simulink model "V4_Modell_Wagen"  (R2022a)
settings: Solver=ode3  StartTime=0.0  StopTime=Zeit(end)  FixedStep=0.00001  RelTol=1e-3
values from neighbouring files (symbols this model uses):
  A = 0.01155    [V4_Parameter_Wagen_St.m]    (also in V4_Parameter_Wagen_Te.m; V4_Parameter_komplett_St.m; V4_Parameter_komplett_Te.m)
  c_W = 0.81    [V4_Parameter_Wagen_St.m]    (also in V4_Parameter_Wagen_Te.m; V4_Parameter_komplett_St.m; V4_Parameter_komplett_Te.m)
  g = 9.81    [V4_Parameter_Wagen_St.m]    (also in V4_Parameter_Wagen_Te.m; V4_Parameter_komplett_St.m; V4_Parameter_komplett_Te.m)
  gamma_rad = gamma_deg * (pi/180)    (= 0.349065850399)    [V4_Parameter_Wagen_St.m]    (also in V4_Parameter_Wagen_Te.m; V4_Parameter_komplett_St.m; V4_Parameter_komplett_Te.m)
  k = (m_Trans + m_ErsatzAntrieb + m_ErsatzRad) / (m_Trans)    [V4_Parameter_Wagen_St.m]    (also in V4_Parameter_Wagen_Te.m; V4_Parameter_komplett_St.m; V4_Parameter_komplett_Te.m)
  k_M = -0.038462    [V4_Parameter_EM.m]    (also in V4_Parameter_Wagen_St.m; V4_Parameter_Wagen_Te.m; V4_Parameter_komplett_St.m; V4_Parameter_komplett_Te.m)
  m_Trans = m_W + 4*m_R    (= 2.157)    [V4_Parameter_Wagen_St.m]    (also in V4_Parameter_Wagen_Te.m = 1.7232; V4_Parameter_komplett_St.m; V4_Parameter_komplett_Te.m = 1.7232)
  mu_R = 0.043    [V4_Parameter_Wagen_St.m]    (also in V4_Parameter_Wagen_Te.m = 0.045; V4_Parameter_komplett_St.m; V4_Parameter_komplett_Te.m = 0.045)
  r_ZR = 25 * (10^(-3))    (= 0.025)    [V4_Parameter_EM.m]    (also in V4_Parameter_Wagen_St.m = 0.021; V4_Parameter_Wagen_Te.m = 0.021; V4_Parameter_komplett_St.m; V4_Parameter_komplett_Te.m)
  rho_L = 1.2    [V4_Parameter_Wagen_St.m]    (also in V4_Parameter_Wagen_Te.m; V4_Parameter_komplett_St.m; V4_Parameter_komplett_Te.m)
settings Model: Creator=bornk  LastModifiedBy=bornk

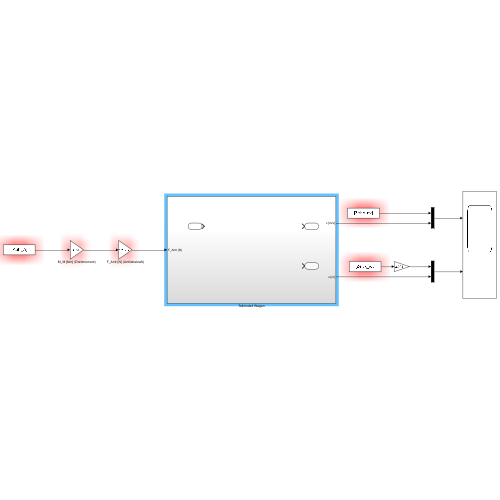
[thumbnail: Simulink's stored preview of the top-level diagram]
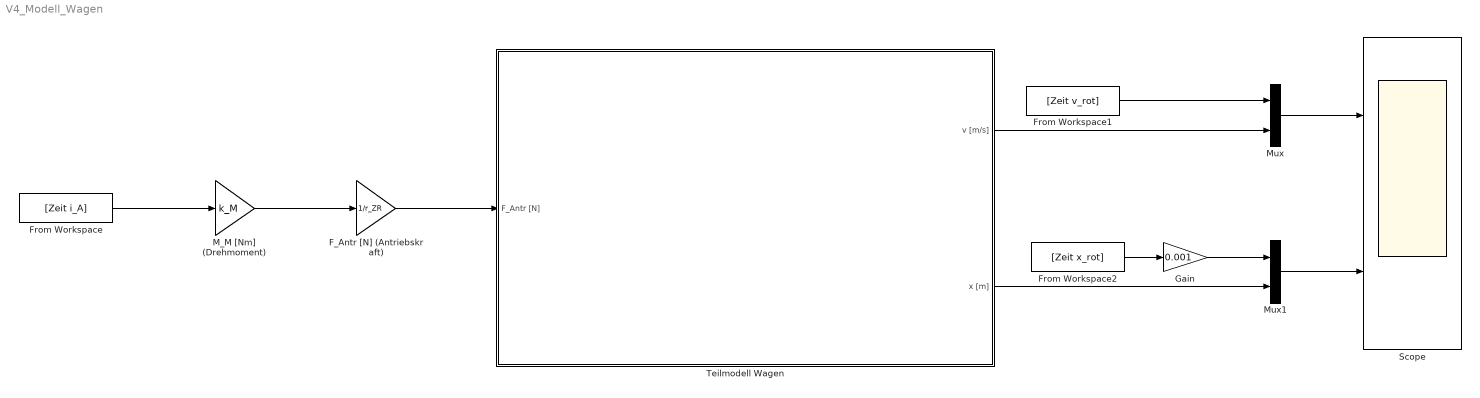
== system V4_Modell_Wagen ==
  F_Antr [N] (Antriebskraft) : Gain  Gain=1/r_ZR
  From Workspace : FromWorkspace  VariableName=[Zeit i_A]
  From Workspace1 : FromWorkspace  VariableName=[Zeit v_rot]
  From Workspace2 : FromWorkspace  VariableName=[Zeit x_rot]
  Gain : Gain  Gain=0.001
  M_M [Nm] (Drehmoment) : Gain  Gain=k_M
  Mux : Mux  Inputs=2
  Mux1 : Mux  Inputs=2
  Scope : Scope  NumInputPorts=2
  Teilmodell Wagen : Subsystem
  wires:
  M_M [Nm] (Drehmoment)/1 -> F_Antr [N] (Antriebskraft)/1
  From Workspace/1 -> M_M [Nm] (Drehmoment)/1
  F_Antr [N] (Antriebskraft)/1 -> Teilmodell Wagen/1(F_Antr [N])
  Teilmodell Wagen/1(v [m/s]) -> Mux/2
  Teilmodell Wagen/2(x [m]) -> Mux1/2
  From Workspace1/1 -> Mux/1
  From Workspace2/1 -> Gain/1
  Gain/1 -> Mux1/1
  Mux/1 -> Scope/1
  Mux1/1 -> Scope/2

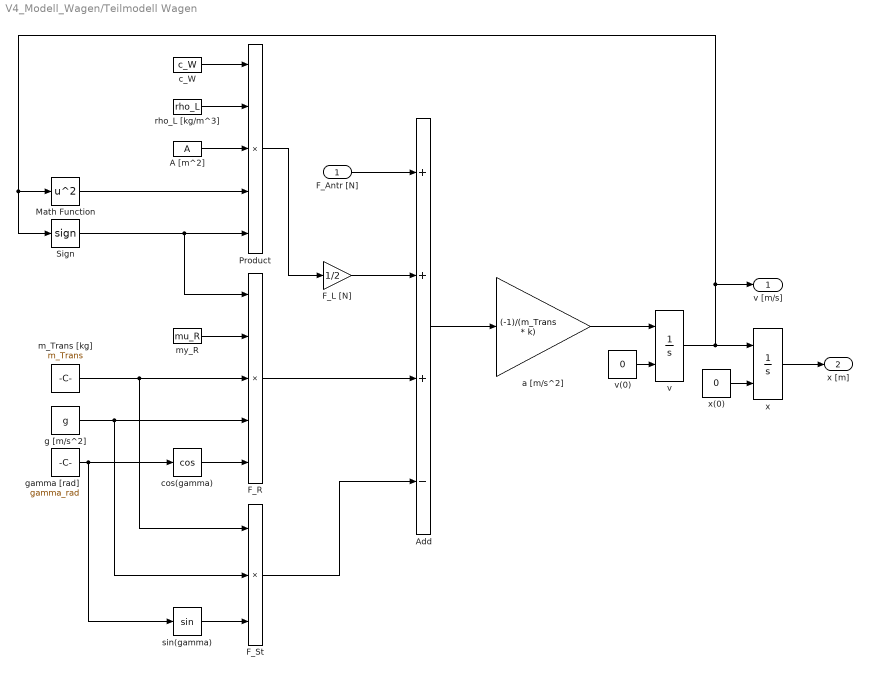
== system V4_Modell_Wagen/Teilmodell Wagen ==
  F_Antr [N] : Inport
  A [m^2] : Constant  Value=A
  Add : Sum  Inputs=+++-
  F_L [N] : Gain  Gain=1/2
  F_R : Product  Inputs=5
  F_St : Product  Inputs=3
  Math Function : Math  Operator=square
  Product : Product  Inputs=5
  Sign : Signum
  a [m/s^2] : Gain  Gain=(-1)/(m_Trans * k)
  c_W : Constant  Value=c_W
  cos(gamma) : Trigonometry  Operator=cos
  g [m/s^2] : Constant  Value=g
  gamma [rad] : Constant  Value=gamma_rad
  m_Trans [kg] : Constant  Value=m_Trans
  my_R : Constant  Value=mu_R
  rho_L [kg/m^3] : Constant  Value=rho_L
  sin(gamma) : Trigonometry
  v : Integrator  InitialConditionSource=external
  v(0) : Constant  Value=0
  x : Integrator  InitialConditionSource=external
  x(0) : Constant  Value=0
  v [m/s] : Outport
  x [m] : Outport  Port=2
  wires:
  F_Antr [N]/1 -> Add/1
  F_L [N]/1 -> Add/2
  Product/1 -> F_L [N]/1
  A [m^2]/1 -> Product/3
  rho_L [kg/m^3]/1 -> Product/2
  c_W/1 -> Product/1
  Sign/1 -> F_R/1, Product/5
  Math Function/1 -> Product/4
  F_R/1 -> Add/3
  my_R/1 -> F_R/2
  m_Trans [kg]/1 -> F_St/1, F_R/3
  g [m/s^2]/1 -> F_St/2, F_R/4
  gamma [rad]/1 -> sin(gamma)/1, cos(gamma)/1
  cos(gamma)/1 -> F_R/5
  sin(gamma)/1 -> F_St/3
  F_St/1 -> Add/4
  Add/1 -> a [m/s^2]/1
  a [m/s^2]/1 -> v/1
  v(0)/1 -> v/2
  v/1 -> v [m/s]/1, Math Function/1, Sign/1, x/1
  x(0)/1 -> x/2
  x/1 -> x [m]/1
